simulink model "twoarea_SOC_henkou"  (R2018b)
settings: Solver=ode3  StartTime=0.0  StopTime=150  FixedStep=0.1  RelTol=1e-3  EnableMultiTasking=on
values from neighbouring files (symbols this model uses):
  f0 = 60    [oneareaSOC.m]
  Ki = 0.1    [oneareaSOC.m]
  Psch = 0    [oneareaSOC.m]
  R = 3    [oneareaSOC.m]
undefined symbols (not defined in the file or in its folder): sigbuilder_block
libraries: simulink_need_slupdate x2
settings Model: Creator=EPESL  LastModifiedBy=EPESL
settings DebuggingCC: UnderSpecifiedDimensionMsg=warning

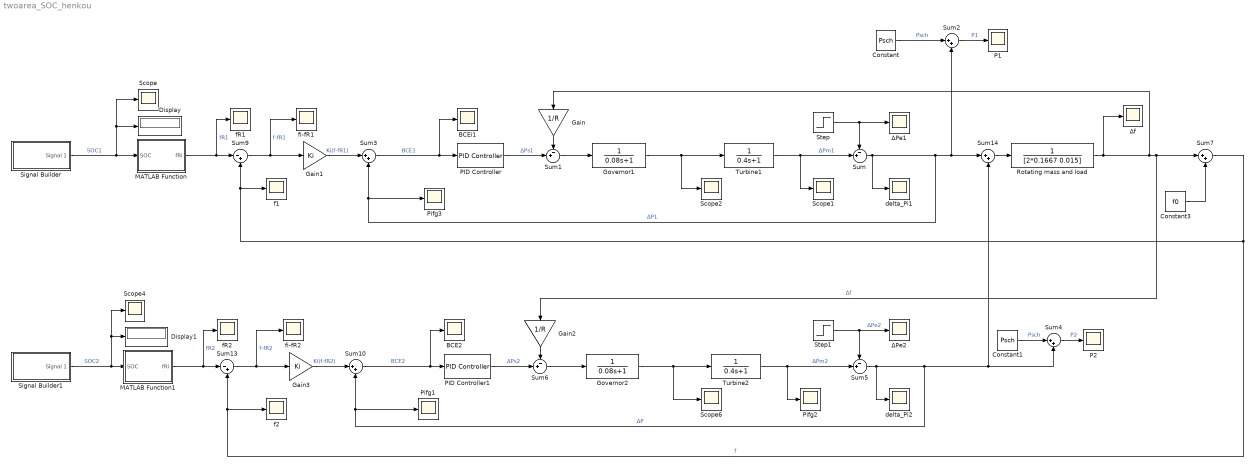
== system twoarea_SOC_henkou ==
  BCE2 : Scope
  BCEi1 : Scope
  Constant : Constant  Value=Psch
  Constant1 : Constant  Value=Psch
  Constant3 : Constant  Value=f0
  Display : Display
  Display1 : Display
  Gain : Gain  Gain=1/R
  Gain1 : Gain  Gain=Ki
  Gain2 : Gain  Gain=1/R
  Gain3 : Gain  Gain=Ki
  Governor1 : TransferFcn  Denominator=[0.08 1]
  Governor2 : TransferFcn  Denominator=[0.08 1]
  MATLAB Function : MATLAB Function  TreatAsAtomicUnit=on
  MATLAB Function1 : MATLAB Function  TreatAsAtomicUnit=on
  P1 : Scope
  P2 : Scope
  PID Controller : simulink_need_slupdate/PID Controller  P=0  I=-0.3  D=0
      settings: SourceProductName=Simulink
  PID Controller1 : simulink_need_slupdate/PID Controller  P=0  I=-0.3  D=0
      settings: SourceProductName=Simulink
  Pifg1 : Scope
  Pifg2 : Scope
  Pifg3 : Scope
  Rotating mass and load : TransferFcn  Denominator=[2*0.1667 0.015]
  Scope{,1..2,4,6} (5 alike) : Scope
  Signal Builder : Subsystem  Tag=STV Subsys  LoadFcn=sigbuilder_block('load');  StartFcn=sigbuilder_block('start');  StopFcn=sigbuilder_block('stop');  ClipboardFcn=sigbuilder_block('clipboard');  mask(Sigbuilder block){tuvar=[0:10]}
      mask help: Simulink:masks:SigbuilderBlock_MD
      mask init:
      | if ~strcmp(get_param(bdroot(gcbh),'SimulationStatus'),'stopped') tuvar = sigbuilder_block('maskInit'); end
      settings: CopyFcn=sigbuilder_block('copy');  DeleteFcn=sigbuilder_block('delete');  ModelCloseFcn=sigbuilder_block('modelClose');  PreSaveFcn=sigbuilder_block('preSave');  PauseFcn=sigbuilder_block('pause');  ContinueFcn=sigbuilder_block('continue');  NameChangeFcn=sigbuilder_block('namechange');  OpenFcn=sigbuilder_block('open',[437.6 199.2 550.4 400 ]);  CloseFcn=sigbuilder_block('close');
      mask Display: plot(0, 0, 100, 100,[2, 2, 32, 32, 2], [68, 8, 8, 68, 68],[32, 2], [38, 38], [32, 19, 2],[53, 60, 44], [32, 17, 17, 2],[16, 16, 31, 31]);txt = getActiveGroup(gcbh);text(2, 100, txt,'verticalAlignment', 'top');
  Signal Builder1 : Subsystem  Tag=STV Subsys  LoadFcn=sigbuilder_block('load');  StartFcn=sigbuilder_block('start');  StopFcn=sigbuilder_block('stop');  ClipboardFcn=sigbuilder_block('clipboard');  mask(Sigbuilder block){tuvar=[0:10]}
      mask help: Simulink:masks:SigbuilderBlock_MD
      mask init:
      | if ~strcmp(get_param(bdroot(gcbh),'SimulationStatus'),'stopped') tuvar = sigbuilder_block('maskInit'); end
      settings: CopyFcn=sigbuilder_block('copy');  DeleteFcn=sigbuilder_block('delete');  ModelCloseFcn=sigbuilder_block('modelClose');  PreSaveFcn=sigbuilder_block('preSave');  PauseFcn=sigbuilder_block('pause');  ContinueFcn=sigbuilder_block('continue');  NameChangeFcn=sigbuilder_block('namechange');  OpenFcn=sigbuilder_block('open',[437.6 199.2 550.4 400 ]);  CloseFcn=sigbuilder_block('close');
      mask Display: plot(0, 0, 100, 100,[2, 2, 32, 32, 2], [68, 8, 8, 68, 68],[32, 2], [38, 38], [32, 19, 2],[53, 60, 44], [32, 17, 17, 2],[16, 16, 31, 31]);txt = getActiveGroup(gcbh);text(2, 100, txt,'verticalAlignment', 'top');
  Step : Step  Time=80  After=0  SampleTime=0
  Step1 : Step  Time=0  After=0  SampleTime=0
  Sum{,1,5..6} (4 alike) : Sum  Inputs=-+|
  Sum{2..4,7,10,14} (6 alike) : Sum  Inputs=|++
  Sum13 : Sum  Inputs=|-+
  Sum9 : Sum  Inputs=|-+
  Turbine1 : TransferFcn  Denominator=[0.4 1]
  Turbine2 : TransferFcn  Denominator=[0.4 1]
  delta_Pi1 : Scope
  delta_Pi2 : Scope
  f1 : Scope
  f2 : Scope
  fR1 : Scope
  fR2 : Scope
  fi-fR1 : Scope
  fi-fR2 : Scope
  ΔPe1 : Scope
  ΔPe2 : Scope
  Δf : Scope
  wires:
  Gain/1 -> Sum1/1
  Step/1 -> ΔPe1/1, Sum/1
  MATLAB Function/1(fRi) -> Sum9/1, fR1/1  "fR1"
  Sum9/1 -> fi-fR1/1, Gain1/1  "f-fR1"
  Rotating mass and load/1 -> Δf/1, Sum7/1, Gain2/1, Gain/1  "Δf"
  Turbine1/1 -> Sum/2, Scope1/1  "ΔPm1"
  Sum1/1 -> Governor1/1
  Governor1/1 -> Scope2/1, Turbine1/1
  Gain1/1 -> Sum3/1  "Ki(f-fR1)"
  Sum3/1 -> BCEi1/1, PID Controller/1  "BCE1"
  PID Controller/1 -> Sum1/2  "ΔPs1"
  Signal Builder/1(Signal 1) -> MATLAB Function/1(SOC), Display/1, Scope/1  "SOC1"
  Sum10/1 -> BCE2/1, PID Controller1/1  "BCE2"
  PID Controller1/1 -> Sum6/2  "ΔPs2"
  Step1/1 -> ΔPe2/1, Sum5/1  "ΔPe2"
  Sum13/1 -> fi-fR2/1, Gain3/1  "f-fR2"
  Sum6/1 -> Governor2/1
  Sum5/1 -> delta_Pi2/1, Sum4/2, Sum14/2, Sum10/2, Pifg1/1  "ΔP"
  Turbine2/1 -> Sum5/2, Pifg2/1  "ΔPm2"
  Gain3/1 -> Sum10/1  "Ki(f-fR2)"
  Governor2/1 -> Scope6/1, Turbine2/1
  Gain2/1 -> Sum6/1
  MATLAB Function1/1(fRi) -> Sum13/1, fR2/1  "fR2"
  Signal Builder1/1(Signal 1) -> Scope4/1, Display1/1, MATLAB Function1/1(SOC)  "SOC2"
  Sum14/1 -> Rotating mass and load/1
  Sum/1 -> delta_Pi1/1, Sum14/1, Sum2/2, Sum3/2, Pifg3/1  "ΔP1"
  Constant/1 -> Sum2/1  "Psch"
  Sum2/1 -> P1/1  "P1"
  Sum4/1 -> P2/1  "P2"
  Constant1/1 -> Sum4/1  "Psch"
  Constant3/1 -> Sum7/2
  Sum7/1 -> f1/1, Sum9/2, f2/1, Sum13/2  "f"

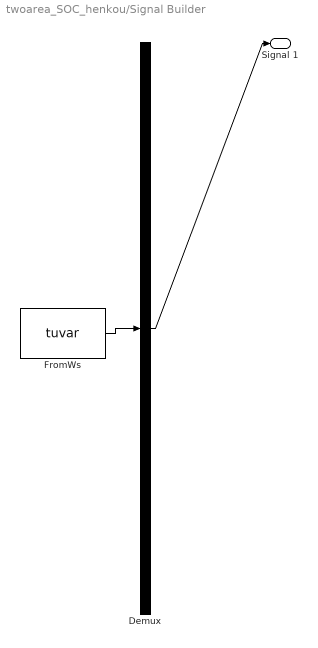
== system twoarea_SOC_henkou/Signal Builder ==
  Demux : Demux  Tag=STV Demux  Outputs=1
  FromWs : FromWorkspace  Tag=STV FromWs  VariableName=tuvar  SampleTime=0
      SigBuilderData=|
      | common.afterFinalStr = 'Extrapolate'
      | common.sampleTime = 0
      | dataSet.timeRange = [0 120]
      | dataSet.name = 'Group 1'
      | sbobj.Groups.Name = 'Group 1'
      | sbobj.Groups.Signals.Name = 'Signal 1'
      | sbobj.Groups.Signals.XData = [0 60 120]
      | sbobj.Groups.Signals.YData = [1 0.5 0.5]
      | sbobj.Groups.TimeRange = [0 120]
  Signal 1 : Outport  Tag=STV Outport
  wires:
  FromWs/1 -> Demux/1
  Demux/1 -> Signal 1/1

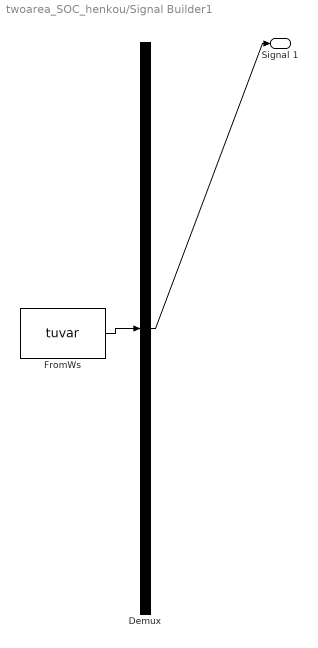
== system twoarea_SOC_henkou/Signal Builder1 ==
  Demux : Demux  Tag=STV Demux  Outputs=1
  FromWs : FromWorkspace  Tag=STV FromWs  VariableName=tuvar  SampleTime=0
      SigBuilderData=|
      | common.afterFinalStr = 'Extrapolate'
      | common.sampleTime = 0
      | dataSet.timeRange = [0 120]
      | dataSet.name = 'Group 1'
      | sbobj.Groups.Name = 'Group 1'
      | sbobj.Groups.Signals.Name = 'Signal 1'
      | sbobj.Groups.Signals.XData = [0 60 120]
      | sbobj.Groups.Signals.YData = [0 0.5 0.5]
      | sbobj.Groups.TimeRange = [0 120]
  Signal 1 : Outport  Tag=STV Outport
  wires:
  FromWs/1 -> Demux/1
  Demux/1 -> Signal 1/1

== matlab function twoarea_SOC_henkou/MATLAB Function1 ==
  data: SOC input; fRi output
function fRi = Func(SOC)

fRi = 59+SOC*(61-59);

== matlab function twoarea_SOC_henkou/MATLAB Function ==
  data: SOC input; fRi output
function fRi = Func(SOC)

fRi = 59+SOC*(61-59);
